simulink model "IEEE30_case"  (R2024b)
settings: Solver=FixedStepAuto  StartTime=0  StopTime=5  FixedStep=1e-7  RelTol=1e-3
values from neighbouring files (symbols this model uses):
  GFL_DFIG_7_C_bus = 0.08    [IEEE30_case_parameters.m]
  GFL_DFIG_7_D_mutual = 2.500000e+3    (= 2500)    [IEEE30_case_parameters.m]
  GFL_DFIG_7_f0 = 60    [IEEE30_case_parameters.m]
  GFL_DFIG_7_gPLLi = 3200    [IEEE30_case_parameters.m]
  GFL_DFIG_7_gPLLp = 650    [IEEE30_case_parameters.m]
  GFL_DFIG_7_H_WT = 0.4    [IEEE30_case_parameters.m]
  GFL_DFIG_7_Hg = 0.8    [IEEE30_case_parameters.m]
  GFL_DFIG_7_Igq_ref = 0    [IEEE30_case_parameters.m]
  GFL_DFIG_7_Ird_ref = 704.45696    [IEEE30_case_parameters.m]
  GFL_DFIG_7_KI_V = -300000    [IEEE30_case_parameters.m]
  GFL_DFIG_7_KP_V = -1000    [IEEE30_case_parameters.m]
  GFL_DFIG_7_Ksh = 1.254300e+4    (= 12543)    [IEEE30_case_parameters.m]
  GFL_DFIG_7_Lg = 0.000483    [IEEE30_case_parameters.m]
  GFL_DFIG_7_Lm_pu = 4    [IEEE30_case_parameters.m]
  GFL_DFIG_7_N = 100    [IEEE30_case_parameters.m]
  GFL_DFIG_7_p = 2    [IEEE30_case_parameters.m]
  GFL_DFIG_7_Pitch = 0    [IEEE30_case_parameters.m]
  GFL_DFIG_7_R = 44    [IEEE30_case_parameters.m]
  GFL_DFIG_7_Rg = 2.000000e-5    (= 2e-05)    [IEEE30_case_parameters.m]
  GFL_DFIG_7_rho = 1.225    [IEEE30_case_parameters.m]
  GFL_DFIG_7_rPLLi = 4500    [IEEE30_case_parameters.m]
  GFL_DFIG_7_rPLLp = 620    [IEEE30_case_parameters.m]
  GFL_DFIG_7_Rs_pu = 0.011    [IEEE30_case_parameters.m]
  GFL_DFIG_7_Sbase = 2.000000e+6    (= 2000000)    [IEEE30_case_parameters.m]
  GFL_DFIG_7_ugq_ref = 0    [IEEE30_case_parameters.m]
  GFL_DFIG_7_usd_ref = 0    [IEEE30_case_parameters.m]
  GFL_DFIG_7_Vbase = 690    [IEEE30_case_parameters.m]
  GFL_DFIG_7_Vdc_ref = 1200    [IEEE30_case_parameters.m]
  GFL_DFIG_7_wind = 12    [IEEE30_case_parameters.m]
  GFL_DFIG_7_wm_ref = 518.184209    [IEEE30_case_parameters.m]
  SG_D_13_D = 0.01056    [IEEE30_case_parameters.m]
  SG_D_13_EnableSaturation = 0    [IEEE30_case_parameters.m]
  SG_D_13_f0 = 60    [IEEE30_case_parameters.m]
  SG_D_13_H = 7.5    [IEEE30_case_parameters.m]
  SG_D_13_K_A = 20    [IEEE30_case_parameters.m]
  SG_D_13_K_E = 1.000000e+1    (= 10)    [IEEE30_case_parameters.m]
  SG_D_13_K_F = 2.363    [IEEE30_case_parameters.m]
  SG_D_13_K_s = 0.5    [IEEE30_case_parameters.m]
  SG_D_13_R_a = 0.001088    [IEEE30_case_parameters.m]
  SG_D_13_S_A = 1    [IEEE30_case_parameters.m]
  SG_D_13_S_B = 0.103    [IEEE30_case_parameters.m]
  SG_D_13_S_N = 10.659857    [IEEE30_case_parameters.m]
  SG_D_13_SpeedPara = 200    [IEEE30_case_parameters.m]
  SG_D_13_T_0 = 0.370163    [IEEE30_case_parameters.m]
  SG_D_13_T_1 = 0.3    [IEEE30_case_parameters.m]
  SG_D_13_T_2 = 0.05    [IEEE30_case_parameters.m]
  SG_D_13_T_3 = 0.02    [IEEE30_case_parameters.m]
  SG_D_13_T_4 = 0.005    [IEEE30_case_parameters.m]
  SG_D_13_T_A = 0.02    [IEEE30_case_parameters.m]
  SG_D_13_T_dd = 8.000000e+0    (= 8)    [IEEE30_case_parameters.m]
  SG_D_13_T_ddd = 0.04    [IEEE30_case_parameters.m]
  SG_D_13_T_E = 0.314    [IEEE30_case_parameters.m]
  SG_D_13_T_F = 0.35    [IEEE30_case_parameters.m]
  SG_D_13_T_qd = 0.8    [IEEE30_case_parameters.m]
  SG_D_13_T_qdd = 0.02    [IEEE30_case_parameters.m]
  SG_D_13_T_speed = 0.1    [IEEE30_case_parameters.m]
  SG_D_13_T_w = 0.5    [IEEE30_case_parameters.m]
  SG_D_13_V_ref = 1.696619    [IEEE30_case_parameters.m]
  SG_D_13_w_ref = 376.991118    [IEEE30_case_parameters.m]
  SG_D_13_x_d = 1.9    [IEEE30_case_parameters.m]
  SG_D_13_x_dd = 0.302    [IEEE30_case_parameters.m]
  SG_D_13_x_ddd = 0.204    [IEEE30_case_parameters.m]
  SG_D_13_x_l = 0.05    [IEEE30_case_parameters.m]
  SG_D_13_x_q = 1.3    [IEEE30_case_parameters.m]
  SG_D_13_x_qd = 0.5    [IEEE30_case_parameters.m]
  SG_D_13_x_qdd = 0.3    [IEEE30_case_parameters.m]
  SG_D_1_D = 0.01056    [IEEE30_case_parameters.m]
  SG_D_1_EnableSaturation = 0    [IEEE30_case_parameters.m]
  SG_D_1_f0 = 60    [IEEE30_case_parameters.m]
  SG_D_1_H = 7.5    [IEEE30_case_parameters.m]
  SG_D_1_K_A = 20    [IEEE30_case_parameters.m]
  SG_D_1_K_E = 1.000000e+1    (= 10)    [IEEE30_case_parameters.m]
  SG_D_1_K_F = 2.363    [IEEE30_case_parameters.m]
  SG_D_1_K_s = 0.5    [IEEE30_case_parameters.m]
  SG_D_1_R_a = 0.001088    [IEEE30_case_parameters.m]
  SG_D_1_S_A = 1    [IEEE30_case_parameters.m]
  SG_D_1_S_B = 0.103    [IEEE30_case_parameters.m]
  SG_D_1_S_N = 10.659857    [IEEE30_case_parameters.m]
  SG_D_1_SpeedPara = 200    [IEEE30_case_parameters.m]
  SG_D_1_T_0 = 0.259812    [IEEE30_case_parameters.m]
  SG_D_1_T_1 = 0.3    [IEEE30_case_parameters.m]
  SG_D_1_T_2 = 0.05    [IEEE30_case_parameters.m]
  SG_D_1_T_3 = 0.02    [IEEE30_case_parameters.m]
  SG_D_1_T_4 = 0.005    [IEEE30_case_parameters.m]
  SG_D_1_T_A = 0.02    [IEEE30_case_parameters.m]
  SG_D_1_T_dd = 8.000000e+0    (= 8)    [IEEE30_case_parameters.m]
  SG_D_1_T_ddd = 0.04    [IEEE30_case_parameters.m]
  SG_D_1_T_E = 0.314    [IEEE30_case_parameters.m]
  SG_D_1_T_F = 0.35    [IEEE30_case_parameters.m]
  SG_D_1_T_qd = 0.8    [IEEE30_case_parameters.m]
  SG_D_1_T_qdd = 0.02    [IEEE30_case_parameters.m]
  SG_D_1_T_speed = 0.1    [IEEE30_case_parameters.m]
  SG_D_1_T_w = 0.5    [IEEE30_case_parameters.m]
  SG_D_1_V_ref = 1.544107    [IEEE30_case_parameters.m]
  SG_D_1_w_ref = 376.991118    [IEEE30_case_parameters.m]
  SG_D_1_x_d = 1.9    [IEEE30_case_parameters.m]
  SG_D_1_x_dd = 0.302    [IEEE30_case_parameters.m]
  SG_D_1_x_ddd = 0.204    [IEEE30_case_parameters.m]
  SG_D_1_x_l = 0.05    [IEEE30_case_parameters.m]
  SG_D_1_x_q = 1.3    [IEEE30_case_parameters.m]
  SG_D_1_x_qd = 0.5    [IEEE30_case_parameters.m]
  SG_D_1_x_qdd = 0.3    [IEEE30_case_parameters.m]
  SG_D_22_D = 0.01056    [IEEE30_case_parameters.m]
  SG_D_22_EnableSaturation = 0    [IEEE30_case_parameters.m]
  SG_D_22_f0 = 60    [IEEE30_case_parameters.m]
  SG_D_22_H = 7.5    [IEEE30_case_parameters.m]
  SG_D_22_K_A = 20    [IEEE30_case_parameters.m]
  SG_D_22_K_E = 1.000000e+1    (= 10)    [IEEE30_case_parameters.m]
  SG_D_22_K_F = 2.363    [IEEE30_case_parameters.m]
  SG_D_22_K_s = 0.5    [IEEE30_case_parameters.m]
  SG_D_22_R_a = 0.001088    [IEEE30_case_parameters.m]
  SG_D_22_S_A = 1    [IEEE30_case_parameters.m]
  SG_D_22_S_B = 0.103    [IEEE30_case_parameters.m]
  SG_D_22_S_N = 10.659857    [IEEE30_case_parameters.m]
  SG_D_22_SpeedPara = 200    [IEEE30_case_parameters.m]
  SG_D_22_T_0 = 0.216121    [IEEE30_case_parameters.m]
  SG_D_22_T_1 = 0.3    [IEEE30_case_parameters.m]
  SG_D_22_T_2 = 0.05    [IEEE30_case_parameters.m]
  SG_D_22_T_3 = 0.02    [IEEE30_case_parameters.m]
  SG_D_22_T_4 = 0.005    [IEEE30_case_parameters.m]
  ... (+126 more)
(part 3 of 27)

== system IEEE30_case/GFL_DFIG_7 ==
  v_d_GFL_DFIG_7 : Inport
  v_q_GFL_DFIG_7 : Inport  Port=2
  Phi_ga_GFL_DFIG_7 : Integrator  InitialCondition=-3.864590758475076e-10
  Phi_gb_GFL_DFIG_7 : Integrator  InitialCondition=0.009328141747306295
  Phi_gc_GFL_DFIG_7 : Integrator  InitialCondition=482731.33548516966
  Phi_ra_GFL_DFIG_7 : Integrator  InitialCondition=2.029121350382751
  Phi_rb_GFL_DFIG_7 : Integrator  InitialCondition=3.675917935843726
  Phi_rc_GFL_DFIG_7 : Integrator  InitialCondition=-6744.715803637379
  Phipllg_GFL_DFIG_7 : Integrator  InitialCondition=0.0
  Phipllr_GFL_DFIG_7 : Integrator  InitialCondition=0.0
  Psi_dr_GFL_DFIG_7 : Integrator  InitialCondition=1.7971026996671524
  Psi_ds_GFL_DFIG_7 : Integrator  InitialCondition=1.7793096036324896
  Psi_qr_GFL_DFIG_7 : Integrator  InitialCondition=0.06414812889743245
  Psi_qs_GFL_DFIG_7 : Integrator  InitialCondition=2.273401543592287e-13
  T_e_GFL_DFIG_7_block : Subsystem
  Turbine_w_GFL_DFIG_7 : Integrator  InitialCondition=259.0921046354467
  V_dc_GFL_DFIG_7 : Integrator  InitialCondition=1200.0
  d_Phi_ga_GFL_DFIG_7_block : Subsystem
  d_Phi_gb_GFL_DFIG_7_block : Subsystem
  d_Phi_gc_GFL_DFIG_7_block : Subsystem
  d_Phi_ra_GFL_DFIG_7_block : Subsystem
  d_Phi_rb_GFL_DFIG_7_block : Subsystem
  d_Phi_rc_GFL_DFIG_7_block : Subsystem
  d_Phipllg_GFL_DFIG_7_block : Subsystem
  d_Phipllr_GFL_DFIG_7_block : Subsystem
  d_Psi_dr_GFL_DFIG_7_block : Subsystem
  d_Psi_ds_GFL_DFIG_7_block : Subsystem
  d_Psi_qr_GFL_DFIG_7_block : Subsystem
  d_Psi_qs_GFL_DFIG_7_block : Subsystem
  d_Turbine_w_GFL_DFIG_7_block : Subsystem
  d_V_dc_GFL_DFIG_7_block : Subsystem
  d_i_gd_GFL_DFIG_7_block : Subsystem
  d_i_gq_GFL_DFIG_7_block : Subsystem
  d_shaft_w_GFL_DFIG_7_block : Subsystem
  d_theta_pllg_GFL_DFIG_7_block : Subsystem
  d_theta_pllr_GFL_DFIG_7_block : Subsystem
  d_w_m_GFL_DFIG_7_block : Subsystem
  i_d_GFL_DFIG_7_block : Subsystem
  i_gd_GFL_DFIG_7 : Integrator  InitialCondition=466.4070874252847
  i_gq_GFL_DFIG_7 : Integrator  InitialCondition=5.309080990232214e-32
  i_q_GFL_DFIG_7_block : Subsystem
  shaft_w_GFL_DFIG_7 : Integrator  InitialCondition=-0.620914212798937
  theta_pllg_GFL_DFIG_7 : Integrator  InitialCondition=0.04628328286195157
  theta_pllr_GFL_DFIG_7 : Integrator  InitialCondition=-1.5245130439329455
  w_m_GFL_DFIG_7 : Integrator  InitialCondition=518.1842092708933
  w_r_GFL_DFIG_7_block : Subsystem
  i_d_GFL_DFIG_7 : Outport
  i_q_GFL_DFIG_7 : Outport  Port=2
  T_e_GFL_DFIG_7 : Outport  Port=3
  w_r_GFL_DFIG_7 : Outport  Port=4
  wires:
  Phipllg_GFL_DFIG_7/1 -> d_theta_pllg_GFL_DFIG_7_block/1(State_Phipllg_GFL_DFIG_7_ae55c)
  d_w_m_GFL_DFIG_7_block/1(Blockout_d_w_m_GFL_DFIG_7_977b5) -> w_m_GFL_DFIG_7/1
  i_gd_GFL_DFIG_7/1 -> d_i_gd_GFL_DFIG_7_block/3(State_i_gd_GFL_DFIG_7_79282), i_q_GFL_DFIG_7_block/1(State_i_gd_GFL_DFIG_7_7f088), i_d_GFL_DFIG_7_block/1(State_i_gd_GFL_DFIG_7_c7c38), d_i_gd_GFL_DFIG_7_block/2(State_i_gd_GFL_DFIG_7_e096c), d_V_dc_GFL_DFIG_7_block/1(State_i_gd_GFL_DFIG_7_47a9f), d_Phi_gb_GFL_DFIG_7_block/1(State_i_gd_GFL_DFIG_7_640f4)
  d_Psi_ds_GFL_DFIG_7_block/1(Blockout_d_Psi_ds_GFL_DFIG_7_0935c) -> Psi_ds_GFL_DFIG_7/1
  Phipllr_GFL_DFIG_7/1 -> d_theta_pllr_GFL_DFIG_7_block/1(State_Phipllr_GFL_DFIG_7_8b535)
  i_d_GFL_DFIG_7_block/1(Blockout_i_d_GFL_DFIG_7_2a8ae) -> i_d_GFL_DFIG_7/1
  d_Psi_qr_GFL_DFIG_7_block/1(Blockout_d_Psi_qr_GFL_DFIG_7_49d19) -> Psi_qr_GFL_DFIG_7/1
  i_q_GFL_DFIG_7_block/1(Blockout_i_q_GFL_DFIG_7_ec3de) -> i_q_GFL_DFIG_7/1
  d_Psi_qs_GFL_DFIG_7_block/1(Blockout_d_Psi_qs_GFL_DFIG_7_2d6b6) -> Psi_qs_GFL_DFIG_7/1
  v_q_GFL_DFIG_7/1 -> d_theta_pllr_GFL_DFIG_7_block/4(Input_v_q_GFL_DFIG_7_cdd0f), d_Phipllr_GFL_DFIG_7_block/3(Input_v_q_GFL_DFIG_7_661f6), d_Psi_qs_GFL_DFIG_7_block/6(Input_v_q_GFL_DFIG_7_1b265), d_theta_pllg_GFL_DFIG_7_block/4(Input_v_q_GFL_DFIG_7_c7c1e), d_Phipllg_GFL_DFIG_7_block/3(Input_v_q_GFL_DFIG_7_4b381), d_Psi_ds_GFL_DFIG_7_block/6(Input_v_q_GFL_DFIG_7_712eb), d_V_dc_GFL_DFIG_7_block/4(Input_v_q_GFL_DFIG_7_3c611), d_V_dc_GFL_DFIG_7_block/9(Input_v_q_GFL_DFIG_7_49107)
  Turbine_w_GFL_DFIG_7/1 -> d_shaft_w_GFL_DFIG_7_block/1(State_Turbine_w_GFL_DFIG_7_fd30f), d_w_m_GFL_DFIG_7_block/1(State_Turbine_w_GFL_DFIG_7_8e651), d_Turbine_w_GFL_DFIG_7_block/5(State_Turbine_w_GFL_DFIG_7_921a6), d_Turbine_w_GFL_DFIG_7_block/6(State_Turbine_w_GFL_DFIG_7_deaae), d_Turbine_w_GFL_DFIG_7_block/4(State_Turbine_w_GFL_DFIG_7_01506), d_Turbine_w_GFL_DFIG_7_block/1(State_Turbine_w_GFL_DFIG_7_f59a7)
  d_V_dc_GFL_DFIG_7_block/1(Blockout_d_V_dc_GFL_DFIG_7_1a7e1) -> V_dc_GFL_DFIG_7/1
  w_r_GFL_DFIG_7_block/1(Blockout_w_r_GFL_DFIG_7_71344) -> w_r_GFL_DFIG_7/1
  theta_pllr_GFL_DFIG_7/1 -> d_theta_pllr_GFL_DFIG_7_block/5(State_theta_pllr_GFL_DFIG_7_76fa6), d_theta_pllr_GFL_DFIG_7_block/3(State_theta_pllr_GFL_DFIG_7_64a08), d_Psi_ds_GFL_DFIG_7_block/7(State_theta_pllr_GFL_DFIG_7_2fe4a), d_Psi_ds_GFL_DFIG_7_block/5(State_theta_pllr_GFL_DFIG_7_d96f9), d_Phipllr_GFL_DFIG_7_block/2(State_theta_pllr_GFL_DFIG_7_673d7), d_Phipllr_GFL_DFIG_7_block/4(State_theta_pllr_GFL_DFIG_7_c3596), i_q_GFL_DFIG_7_block/10(State_theta_pllr_GFL_DFIG_7_b0808), d_Psi_qs_GFL_DFIG_7_block/5(State_theta_pllr_GFL_DFIG_7_5db89), d_Psi_qs_GFL_DFIG_7_block/7(State_theta_pllr_GFL_DFIG_7_ab88b), i_d_GFL_DFIG_7_block/7(State_theta_pllr_GFL_DFIG_7_79db7), i_d_GFL_DFIG_7_block/10(State_theta_pllr_GFL_DFIG_7_e04ad), i_q_GFL_DFIG_7_block/7(State_theta_pllr_GFL_DFIG_7_9bdbf)
  V_dc_GFL_DFIG_7/1 -> d_Phi_gc_GFL_DFIG_7_block/1(State_V_dc_GFL_DFIG_7_30c65), d_i_gd_GFL_DFIG_7_block/4(State_V_dc_GFL_DFIG_7_27989), d_Phi_gb_GFL_DFIG_7_block/2(State_V_dc_GFL_DFIG_7_6d222), d_V_dc_GFL_DFIG_7_block/34(State_V_dc_GFL_DFIG_7_49932)
  Phi_ga_GFL_DFIG_7/1 -> d_i_gq_GFL_DFIG_7_block/1(State_Phi_ga_GFL_DFIG_7_1abf4)
  T_e_GFL_DFIG_7_block/1(Blockout_T_e_GFL_DFIG_7_ea981) -> T_e_GFL_DFIG_7/1
  Phi_gb_GFL_DFIG_7/1 -> d_i_gd_GFL_DFIG_7_block/1(State_Phi_gb_GFL_DFIG_7_1acd8)
  d_Phipllg_GFL_DFIG_7_block/1(Blockout_d_Phipllg_GFL_DFIG_7_57d75) -> Phipllg_GFL_DFIG_7/1
  theta_pllg_GFL_DFIG_7/1 -> d_theta_pllg_GFL_DFIG_7_block/3(State_theta_pllg_GFL_DFIG_7_2f4db), d_theta_pllg_GFL_DFIG_7_block/5(State_theta_pllg_GFL_DFIG_7_b3c0b), i_d_GFL_DFIG_7_block/2(State_theta_pllg_GFL_DFIG_7_3c4e6), i_d_GFL_DFIG_7_block/4(State_theta_pllg_GFL_DFIG_7_99cce), i_q_GFL_DFIG_7_block/2(State_theta_pllg_GFL_DFIG_7_b67ea), i_q_GFL_DFIG_7_block/4(State_theta_pllg_GFL_DFIG_7_36f0a), d_Phipllg_GFL_DFIG_7_block/4(State_theta_pllg_GFL_DFIG_7_1f5b3), d_Phipllg_GFL_DFIG_7_block/2(State_theta_pllg_GFL_DFIG_7_d7c88), d_V_dc_GFL_DFIG_7_block/3(State_theta_pllg_GFL_DFIG_7_c67a2), d_V_dc_GFL_DFIG_7_block/5(State_theta_pllg_GFL_DFIG_7_35391), d_V_dc_GFL_DFIG_7_block/8(State_theta_pllg_GFL_DFIG_7_002e2), d_V_dc_GFL_DFIG_7_block/10(State_theta_pllg_GFL_DFIG_7_66e51)
  i_gq_GFL_DFIG_7/1 -> d_i_gq_GFL_DFIG_7_block/3(State_i_gq_GFL_DFIG_7_5be6d), d_i_gq_GFL_DFIG_7_block/2(State_i_gq_GFL_DFIG_7_3f6ab), d_Phi_ga_GFL_DFIG_7_block/1(State_i_gq_GFL_DFIG_7_ca300), i_q_GFL_DFIG_7_block/3(State_i_gq_GFL_DFIG_7_cf5eb), d_V_dc_GFL_DFIG_7_block/6(State_i_gq_GFL_DFIG_7_793b6), i_d_GFL_DFIG_7_block/3(State_i_gq_GFL_DFIG_7_12231)
  d_Phipllr_GFL_DFIG_7_block/1(Blockout_d_Phipllr_GFL_DFIG_7_3fa24) -> Phipllr_GFL_DFIG_7/1
  Psi_qs_GFL_DFIG_7/1 -> T_e_GFL_DFIG_7_block/4(State_Psi_qs_GFL_DFIG_7_92c6b), T_e_GFL_DFIG_7_block/8(State_Psi_qs_GFL_DFIG_7_3687d), d_Psi_dr_GFL_DFIG_7_block/3(State_Psi_qs_GFL_DFIG_7_a7547), d_Psi_qr_GFL_DFIG_7_block/16(State_Psi_qs_GFL_DFIG_7_c351a), i_d_GFL_DFIG_7_block/9(State_Psi_qs_GFL_DFIG_7_a1324), d_Phi_rb_GFL_DFIG_7_block/4(State_Psi_qs_GFL_DFIG_7_57503), d_Phi_rb_GFL_DFIG_7_block/6(State_Psi_qs_GFL_DFIG_7_e35cc), i_q_GFL_DFIG_7_block/9(State_Psi_qs_GFL_DFIG_7_79723), d_w_m_GFL_DFIG_7_block/7(State_Psi_qs_GFL_DFIG_7_716ac), d_w_m_GFL_DFIG_7_block/11(State_Psi_qs_GFL_DFIG_7_6b007), d_Psi_ds_GFL_DFIG_7_block/1(State_Psi_qs_GFL_DFIG_7_b4caa), d_Psi_qr_GFL_DFIG_7_block/8(State_Psi_qs_GFL_DFIG_7_981a4), d_Psi_qr_GFL_DFIG_7_block/12(State_Psi_qs_GFL_DFIG_7_b24c8), d_Psi_qr_GFL_DFIG_7_block/14(State_Psi_qs_GFL_DFIG_7_c0308), d_Psi_qs_GFL_DFIG_7_block/3(State_Psi_qs_GFL_DFIG_7_b8433), d_V_dc_GFL_DFIG_7_block/30(State_Psi_qs_GFL_DFIG_7_44146), d_V_dc_GFL_DFIG_7_block/32(State_Psi_qs_GFL_DFIG_7_97bd8), d_V_dc_GFL_DFIG_7_block/28(State_Psi_qs_GFL_DFIG_7_f7902), d_V_dc_GFL_DFIG_7_block/20(State_Psi_qs_GFL_DFIG_7_fde33), d_V_dc_GFL_DFIG_7_block/15(State_Psi_qs_GFL_DFIG_7_f70b4)
  d_Phi_gb_GFL_DFIG_7_block/1(Blockout_d_Phi_gb_GFL_DFIG_7_12bfd) -> Phi_gb_GFL_DFIG_7/1
  d_Phi_gc_GFL_DFIG_7_block/1(Blockout_d_Phi_gc_GFL_DFIG_7_e7a32) -> Phi_gc_GFL_DFIG_7/1
  d_Phi_ga_GFL_DFIG_7_block/1(Blockout_d_Phi_ga_GFL_DFIG_7_179fc) -> Phi_ga_GFL_DFIG_7/1
  Psi_dr_GFL_DFIG_7/1 -> d_Psi_dr_GFL_DFIG_7_block/9(State_Psi_dr_GFL_DFIG_7_ac80b), d_Psi_dr_GFL_DFIG_7_block/7(State_Psi_dr_GFL_DFIG_7_f20f7), d_V_dc_GFL_DFIG_7_block/22(State_Psi_dr_GFL_DFIG_7_978cf), d_V_dc_GFL_DFIG_7_block/17(State_Psi_dr_GFL_DFIG_7_0acea), d_V_dc_GFL_DFIG_7_block/11(State_Psi_dr_GFL_DFIG_7_6e653), T_e_GFL_DFIG_7_block/1(State_Psi_dr_GFL_DFIG_7_7f61d), T_e_GFL_DFIG_7_block/5(State_Psi_dr_GFL_DFIG_7_e7cd2), i_d_GFL_DFIG_7_block/5(State_Psi_dr_GFL_DFIG_7_47f96), d_Phi_ra_GFL_DFIG_7_block/1(State_Psi_dr_GFL_DFIG_7_3e6d6), i_q_GFL_DFIG_7_block/5(State_Psi_dr_GFL_DFIG_7_f818d), d_Psi_qr_GFL_DFIG_7_block/5(State_Psi_dr_GFL_DFIG_7_851ca), d_Psi_qr_GFL_DFIG_7_block/2(State_Psi_dr_GFL_DFIG_7_54fa3), d_Psi_ds_GFL_DFIG_7_block/2(State_Psi_dr_GFL_DFIG_7_0949a), d_w_m_GFL_DFIG_7_block/8(State_Psi_dr_GFL_DFIG_7_9aecf), d_w_m_GFL_DFIG_7_block/4(State_Psi_dr_GFL_DFIG_7_d08b0)
  d_theta_pllg_GFL_DFIG_7_block/1(Blockout_d_theta_pllg_GFL_DFIG_7_9b0fc) -> theta_pllg_GFL_DFIG_7/1
  Phi_gc_GFL_DFIG_7/1 -> d_i_gd_GFL_DFIG_7_block/5(State_Phi_gc_GFL_DFIG_7_ffb8d), d_Phi_gb_GFL_DFIG_7_block/3(State_Phi_gc_GFL_DFIG_7_b7107)
  d_theta_pllr_GFL_DFIG_7_block/1(Blockout_d_theta_pllr_GFL_DFIG_7_2facc) -> theta_pllr_GFL_DFIG_7/1
  d_Phi_rb_GFL_DFIG_7_block/1(Blockout_d_Phi_rb_GFL_DFIG_7_7ae6c) -> Phi_rb_GFL_DFIG_7/1
  d_Psi_dr_GFL_DFIG_7_block/1(Blockout_d_Psi_dr_GFL_DFIG_7_75b07) -> Psi_dr_GFL_DFIG_7/1
  d_Phi_rc_GFL_DFIG_7_block/1(Blockout_d_Phi_rc_GFL_DFIG_7_aa447) -> Phi_rc_GFL_DFIG_7/1
  Phi_rc_GFL_DFIG_7/1 -> d_Psi_qr_GFL_DFIG_7_block/9(State_Phi_rc_GFL_DFIG_7_1cf80), d_Phi_rb_GFL_DFIG_7_block/1(State_Phi_rc_GFL_DFIG_7_bc2c9), d_V_dc_GFL_DFIG_7_block/25(State_Phi_rc_GFL_DFIG_7_c7d1c)
  d_Phi_ra_GFL_DFIG_7_block/1(Blockout_d_Phi_ra_GFL_DFIG_7_b9bb2) -> Phi_ra_GFL_DFIG_7/1
  d_Turbine_w_GFL_DFIG_7_block/1(Blockout_d_Turbine_w_GFL_DFIG_7_37f45) -> Turbine_w_GFL_DFIG_7/1
  v_d_GFL_DFIG_7/1 -> d_theta_pllr_GFL_DFIG_7_block/2(Input_v_d_GFL_DFIG_7_57b0c), d_Phipllr_GFL_DFIG_7_block/1(Input_v_d_GFL_DFIG_7_0a8be), d_theta_pllg_GFL_DFIG_7_block/2(Input_v_d_GFL_DFIG_7_973c5), d_Phipllg_GFL_DFIG_7_block/1(Input_v_d_GFL_DFIG_7_9bb07), d_Psi_ds_GFL_DFIG_7_block/4(Input_v_d_GFL_DFIG_7_61464), d_Psi_qs_GFL_DFIG_7_block/4(Input_v_d_GFL_DFIG_7_b1351), d_V_dc_GFL_DFIG_7_block/2(Input_v_d_GFL_DFIG_7_58356), d_V_dc_GFL_DFIG_7_block/7(Input_v_d_GFL_DFIG_7_bbd62)
  w_m_GFL_DFIG_7/1 -> d_Psi_dr_GFL_DFIG_7_block/1(State_w_m_GFL_DFIG_7_ede24), d_Psi_dr_GFL_DFIG_7_block/6(State_w_m_GFL_DFIG_7_c0fab), w_r_GFL_DFIG_7_block/1(State_w_m_GFL_DFIG_7_cf772), d_V_dc_GFL_DFIG_7_block/33(State_w_m_GFL_DFIG_7_46811), d_V_dc_GFL_DFIG_7_block/26(State_w_m_GFL_DFIG_7_35e3b), d_V_dc_GFL_DFIG_7_block/21(State_w_m_GFL_DFIG_7_73a6c), d_V_dc_GFL_DFIG_7_block/13(State_w_m_GFL_DFIG_7_6ca23), d_Psi_qr_GFL_DFIG_7_block/10(State_w_m_GFL_DFIG_7_509a1), d_Phi_rc_GFL_DFIG_7_block/1(State_w_m_GFL_DFIG_7_b5946), d_Psi_qr_GFL_DFIG_7_block/6(State_w_m_GFL_DFIG_7_7741f), d_Psi_qr_GFL_DFIG_7_block/1(State_w_m_GFL_DFIG_7_5fc1b), d_shaft_w_GFL_DFIG_7_block/2(State_w_m_GFL_DFIG_7_93de0), d_w_m_GFL_DFIG_7_block/2(State_w_m_GFL_DFIG_7_dfde2), d_Turbine_w_GFL_DFIG_7_block/2(State_w_m_GFL_DFIG_7_7a0a3), d_Psi_qr_GFL_DFIG_7_block/17(State_w_m_GFL_DFIG_7_084b2), d_Phi_rb_GFL_DFIG_7_block/2(State_w_m_GFL_DFIG_7_5425d)
  Psi_qr_GFL_DFIG_7/1 -> d_Psi_dr_GFL_DFIG_7_block/2(State_Psi_qr_GFL_DFIG_7_b0873), d_Psi_dr_GFL_DFIG_7_block/5(State_Psi_qr_GFL_DFIG_7_8feb7), T_e_GFL_DFIG_7_block/7(State_Psi_qr_GFL_DFIG_7_aa7be), T_e_GFL_DFIG_7_block/3(State_Psi_qr_GFL_DFIG_7_3f5fe), d_Psi_qs_GFL_DFIG_7_block/2(State_Psi_qr_GFL_DFIG_7_e0b4f), d_w_m_GFL_DFIG_7_block/6(State_Psi_qr_GFL_DFIG_7_240a6), i_q_GFL_DFIG_7_block/8(State_Psi_qr_GFL_DFIG_7_bf209), d_w_m_GFL_DFIG_7_block/10(State_Psi_qr_GFL_DFIG_7_28155), i_d_GFL_DFIG_7_block/8(State_Psi_qr_GFL_DFIG_7_2c5a7), d_V_dc_GFL_DFIG_7_block/14(State_Psi_qr_GFL_DFIG_7_2b0e8), d_V_dc_GFL_DFIG_7_block/19(State_Psi_qr_GFL_DFIG_7_f1f75), d_V_dc_GFL_DFIG_7_block/29(State_Psi_qr_GFL_DFIG_7_e69a0), d_Psi_qr_GFL_DFIG_7_block/7(State_Psi_qr_GFL_DFIG_7_c4d86), d_Psi_qr_GFL_DFIG_7_block/13(State_Psi_qr_GFL_DFIG_7_7bb62), d_Phi_rb_GFL_DFIG_7_block/5(State_Psi_qr_GFL_DFIG_7_e4388)
  Psi_ds_GFL_DFIG_7/1 -> d_Psi_dr_GFL_DFIG_7_block/8(State_Psi_ds_GFL_DFIG_7_ccb41), d_Psi_dr_GFL_DFIG_7_block/10(State_Psi_ds_GFL_DFIG_7_652d4), T_e_GFL_DFIG_7_block/6(State_Psi_ds_GFL_DFIG_7_ef1b2), T_e_GFL_DFIG_7_block/2(State_Psi_ds_GFL_DFIG_7_93139), d_Phi_ra_GFL_DFIG_7_block/2(State_Psi_ds_GFL_DFIG_7_9adb5), d_w_m_GFL_DFIG_7_block/5(State_Psi_ds_GFL_DFIG_7_b9ddc), i_q_GFL_DFIG_7_block/6(State_Psi_ds_GFL_DFIG_7_97cbe), d_w_m_GFL_DFIG_7_block/9(State_Psi_ds_GFL_DFIG_7_7aea2), i_d_GFL_DFIG_7_block/6(State_Psi_ds_GFL_DFIG_7_8722f), d_Phi_rb_GFL_DFIG_7_block/3(State_Psi_ds_GFL_DFIG_7_7a16b), d_V_dc_GFL_DFIG_7_block/12(State_Psi_ds_GFL_DFIG_7_832af), d_V_dc_GFL_DFIG_7_block/18(State_Psi_ds_GFL_DFIG_7_692c3), d_V_dc_GFL_DFIG_7_block/23(State_Psi_ds_GFL_DFIG_7_2e09c), d_V_dc_GFL_DFIG_7_block/31(State_Psi_ds_GFL_DFIG_7_a0019), d_V_dc_GFL_DFIG_7_block/27(State_Psi_ds_GFL_DFIG_7_dee5b), d_Psi_qs_GFL_DFIG_7_block/1(State_Psi_ds_GFL_DFIG_7_90de9), d_Psi_ds_GFL_DFIG_7_block/3(State_Psi_ds_GFL_DFIG_7_d7878), d_Psi_qr_GFL_DFIG_7_block/3(State_Psi_ds_GFL_DFIG_7_18bf4), d_Psi_qr_GFL_DFIG_7_block/11(State_Psi_ds_GFL_DFIG_7_e95d8), d_Psi_qr_GFL_DFIG_7_block/15(State_Psi_ds_GFL_DFIG_7_fa3e8)
  shaft_w_GFL_DFIG_7/1 -> d_w_m_GFL_DFIG_7_block/3(State_shaft_w_GFL_DFIG_7_e1a06), d_Turbine_w_GFL_DFIG_7_block/3(State_shaft_w_GFL_DFIG_7_53793)
  Phi_ra_GFL_DFIG_7/1 -> d_Psi_dr_GFL_DFIG_7_block/4(State_Phi_ra_GFL_DFIG_7_e382b), d_V_dc_GFL_DFIG_7_block/16(State_Phi_ra_GFL_DFIG_7_71e34)
  Phi_rb_GFL_DFIG_7/1 -> d_Psi_qr_GFL_DFIG_7_block/4(State_Phi_rb_GFL_DFIG_7_b6830), d_V_dc_GFL_DFIG_7_block/24(State_Phi_rb_GFL_DFIG_7_e2f9d)
  d_i_gd_GFL_DFIG_7_block/1(Blockout_d_i_gd_GFL_DFIG_7_cd2cb) -> i_gd_GFL_DFIG_7/1
  d_i_gq_GFL_DFIG_7_block/1(Blockout_d_i_gq_GFL_DFIG_7_79c3a) -> i_gq_GFL_DFIG_7/1
  d_shaft_w_GFL_DFIG_7_block/1(Blockout_d_shaft_w_GFL_DFIG_7_0b709) -> shaft_w_GFL_DFIG_7/1

== system IEEE30_case/SG_D_1 ==
  v_d_SG_D_1 : Inport
  v_q_SG_D_1 : Inport  Port=2
  E_fd_SG_D_1 : Integrator  InitialCondition=1.0882132920517957
  Px_1_SG_D_1 : Integrator  InitialCondition=0.0
  Px_2_SG_D_1 : Integrator  InitialCondition=0.0
  Px_3_SG_D_1 : Integrator  InitialCondition=-1.2192692551246703e-31
  R_f_SG_D_1 : Integrator  InitialCondition=7.346994311766839
  T_e_SG_D_1_block : Subsystem
  T_m_SG_D_1 : Integrator  InitialCondition=0.2598115405337171
  V_f_SG_D_1 : Integrator  InitialCondition=10.882132920517959
  d_E_fd_SG_D_1_block : Subsystem
  d_Px_1_SG_D_1_block : Subsystem
  d_Px_2_SG_D_1_block : Subsystem
  d_Px_3_SG_D_1_block : Subsystem
  d_R_f_SG_D_1_block : Subsystem
  d_T_m_SG_D_1_block : Subsystem
  d_V_f_SG_D_1_block : Subsystem
  d_psi_1d_SG_D_1_block : Subsystem
  d_psi_d_SG_D_1_block : Subsystem
  d_psi_fd_SG_D_1_block : Subsystem
  d_psi_gq_SG_D_1_block : Subsystem
  d_psi_kq_SG_D_1_block : Subsystem
  d_psi_q_SG_D_1_block : Subsystem
  d_theta_SG_D_1_block : Subsystem
  d_w_SG_D_1_block : Subsystem
  i_d_SG_D_1_block : Subsystem
  i_q_SG_D_1_block : Subsystem
  psi_1d_SG_D_1 : Integrator  InitialCondition=0.950191905636144
  psi_d_SG_D_1 : Integrator  InitialCondition=0.9464615978951803
  psi_fd_SG_D_1 : Integrator  InitialCondition=0.9689926566506003
  psi_gq_SG_D_1 : Integrator  InitialCondition=0.1991943191066703
  psi_kq_SG_D_1 : Integrator  InitialCondition=-0.31124112360417233
  psi_q_SG_D_1 : Integrator  InitialCondition=-0.3236907685483392
  theta_SG_D_1 : Integrator  InitialCondition=0.32954188376716115
  theta_SG_D_1_out_block : Subsystem
  w_SG_D_1 : Integrator  InitialCondition=376.99111843077515
  w_SG_D_1_out_block : Subsystem
  i_d_SG_D_1 : Outport
  i_q_SG_D_1 : Outport  Port=2
  T_e_SG_D_1 : Outport  Port=3
  w_SG_D_1_out : Outport  Port=4
  theta_SG_D_1_out : Outport  Port=5
  wires:
  d_theta_SG_D_1_block/1(Blockout_d_theta_SG_D_1_b4601) -> theta_SG_D_1/1
  d_Px_1_SG_D_1_block/1(Blockout_d_Px_1_SG_D_1_1380a) -> Px_1_SG_D_1/1
  V_f_SG_D_1/1 -> d_V_f_SG_D_1_block/14(State_V_f_SG_D_1_2c940), d_E_fd_SG_D_1_block/2(State_V_f_SG_D_1_4243a)
  psi_kq_SG_D_1/1 -> d_psi_q_SG_D_1_block/2(State_psi_kq_SG_D_1_f77dd), d_psi_gq_SG_D_1_block/3(State_psi_kq_SG_D_1_13d6b), d_psi_gq_SG_D_1_block/5(State_psi_kq_SG_D_1_4933d), d_psi_kq_SG_D_1_block/4(State_psi_kq_SG_D_1_b2a24), d_psi_kq_SG_D_1_block/2(State_psi_kq_SG_D_1_f6edb), d_V_f_SG_D_1_block/10(State_psi_kq_SG_D_1_e81ac), i_d_SG_D_1_block/2(State_psi_kq_SG_D_1_4ef53), d_psi_gq_SG_D_1_block/8(State_psi_kq_SG_D_1_372ae), i_q_SG_D_1_block/2(State_psi_kq_SG_D_1_e6fa4), T_e_SG_D_1_block/3(State_psi_kq_SG_D_1_16b29), d_w_SG_D_1_block/5(State_psi_kq_SG_D_1_2014b)
  w_SG_D_1_out_block/1(Blockout_w_SG_D_1_out_e1973) -> w_SG_D_1_out/1
  w_SG_D_1/1 -> d_psi_d_SG_D_1_block/9(State_w_SG_D_1_d2cfd), d_w_SG_D_1_block/1(State_w_SG_D_1_7370e), d_psi_q_SG_D_1_block/9(State_w_SG_D_1_948ae), d_V_f_SG_D_1_block/8(State_w_SG_D_1_25f13), d_T_m_SG_D_1_block/1(State_w_SG_D_1_e56b0), d_Px_1_SG_D_1_block/2(State_w_SG_D_1_e905d), d_Px_2_SG_D_1_block/4(State_w_SG_D_1_34181), d_Px_3_SG_D_1_block/6(State_w_SG_D_1_e8e94), d_V_f_SG_D_1_block/13(State_w_SG_D_1_84be6), w_SG_D_1_out_block/1(State_w_SG_D_1_f54e8), d_theta_SG_D_1_block/1(State_w_SG_D_1_25fe5)
  d_T_m_SG_D_1_block/1(Blockout_d_T_m_SG_D_1_12514) -> T_m_SG_D_1/1
  d_Px_2_SG_D_1_block/1(Blockout_d_Px_2_SG_D_1_8ee22) -> Px_2_SG_D_1/1
  d_Px_3_SG_D_1_block/1(Blockout_d_Px_3_SG_D_1_3bf99) -> Px_3_SG_D_1/1
  psi_gq_SG_D_1/1 -> d_psi_q_SG_D_1_block/1(State_psi_gq_SG_D_1_26e24), d_psi_gq_SG_D_1_block/1(State_psi_gq_SG_D_1_332f7), d_psi_gq_SG_D_1_block/2(State_psi_gq_SG_D_1_b0dac), d_w_SG_D_1_block/4(State_psi_gq_SG_D_1_ce49a), d_psi_kq_SG_D_1_block/1(State_psi_gq_SG_D_1_66a42), d_V_f_SG_D_1_block/9(State_psi_gq_SG_D_1_d56db), d_psi_kq_SG_D_1_block/3(State_psi_gq_SG_D_1_3bf06), i_d_SG_D_1_block/1(State_psi_gq_SG_D_1_10f28), d_psi_gq_SG_D_1_block/7(State_psi_gq_SG_D_1_3b2a6), d_psi_gq_SG_D_1_block/4(State_psi_gq_SG_D_1_2cb53), i_q_SG_D_1_block/1(State_psi_gq_SG_D_1_d4375), T_e_SG_D_1_block/2(State_psi_gq_SG_D_1_a6910)
  psi_fd_SG_D_1/1 -> d_psi_fd_SG_D_1_block/2(State_psi_fd_SG_D_1_c7574), d_psi_fd_SG_D_1_block/4(State_psi_fd_SG_D_1_fe3bf), d_psi_fd_SG_D_1_block/7(State_psi_fd_SG_D_1_1eed0), d_psi_d_SG_D_1_block/3(State_psi_fd_SG_D_1_f658e), d_psi_1d_SG_D_1_block/2(State_psi_fd_SG_D_1_697dc), i_d_SG_D_1_block/7(State_psi_fd_SG_D_1_0507a), d_psi_1d_SG_D_1_block/5(State_psi_fd_SG_D_1_a7ee9), i_q_SG_D_1_block/7(State_psi_fd_SG_D_1_d5158), T_e_SG_D_1_block/8(State_psi_fd_SG_D_1_a9978), d_w_SG_D_1_block/10(State_psi_fd_SG_D_1_cb4ff), d_V_f_SG_D_1_block/6(State_psi_fd_SG_D_1_18250), d_psi_fd_SG_D_1_block/10(State_psi_fd_SG_D_1_e31c3)
  T_m_SG_D_1/1 -> d_T_m_SG_D_1_block/2(State_T_m_SG_D_1_eb6d8), d_w_SG_D_1_block/2(State_T_m_SG_D_1_0f890)
  v_d_SG_D_1/1 -> d_psi_d_SG_D_1_block/4(Input_v_d_SG_D_1_95be5), d_psi_q_SG_D_1_block/4(Input_v_d_SG_D_1_1c698)
  v_q_SG_D_1/1 -> d_psi_d_SG_D_1_block/6(Input_v_q_SG_D_1_f5767), d_psi_q_SG_D_1_block/6(Input_v_q_SG_D_1_e75ba)
  Px_1_SG_D_1/1 -> d_Px_1_SG_D_1_block/1(State_Px_1_SG_D_1_b81ac), d_Px_3_SG_D_1_block/5(State_Px_1_SG_D_1_665ee), d_Px_3_SG_D_1_block/4(State_Px_1_SG_D_1_64472), d_Px_2_SG_D_1_block/3(State_Px_1_SG_D_1_3856c), d_Px_2_SG_D_1_block/2(State_Px_1_SG_D_1_ae78a)
  Px_2_SG_D_1/1 -> d_Px_2_SG_D_1_block/1(State_Px_2_SG_D_1_7ad78), d_Px_3_SG_D_1_block/2(State_Px_2_SG_D_1_d9b49), d_Px_3_SG_D_1_block/3(State_Px_2_SG_D_1_ab48e)
  theta_SG_D_1/1 -> d_psi_d_SG_D_1_block/5(State_theta_SG_D_1_3e828), d_psi_d_SG_D_1_block/7(State_theta_SG_D_1_93c49), d_psi_q_SG_D_1_block/5(State_theta_SG_D_1_9525e), i_d_SG_D_1_block/4(State_theta_SG_D_1_e11c7), i_d_SG_D_1_block/8(State_theta_SG_D_1_02fe0), i_q_SG_D_1_block/4(State_theta_SG_D_1_9797a), i_q_SG_D_1_block/8(State_theta_SG_D_1_8458a), d_psi_q_SG_D_1_block/7(State_theta_SG_D_1_5ff34), theta_SG_D_1_out_block/1(State_theta_SG_D_1_a2930)
  d_E_fd_SG_D_1_block/1(Blockout_d_E_fd_SG_D_1_3912e) -> E_fd_SG_D_1/1
  psi_1d_SG_D_1/1 -> d_psi_fd_SG_D_1_block/5(State_psi_1d_SG_D_1_b3018), d_psi_fd_SG_D_1_block/8(State_psi_1d_SG_D_1_10652), d_psi_fd_SG_D_1_block/3(State_psi_1d_SG_D_1_1742e), d_psi_d_SG_D_1_block/1(State_psi_1d_SG_D_1_5396e), d_psi_1d_SG_D_1_block/1(State_psi_1d_SG_D_1_acde6), d_psi_1d_SG_D_1_block/3(State_psi_1d_SG_D_1_d153a), i_q_SG_D_1_block/5(State_psi_1d_SG_D_1_a42f8), d_V_f_SG_D_1_block/4(State_psi_1d_SG_D_1_39760), T_e_SG_D_1_block/6(State_psi_1d_SG_D_1_d6542), i_d_SG_D_1_block/5(State_psi_1d_SG_D_1_3ebc3), d_w_SG_D_1_block/8(State_psi_1d_SG_D_1_f2003)
  psi_q_SG_D_1/1 -> d_psi_d_SG_D_1_block/8(State_psi_q_SG_D_1_efd17), d_psi_q_SG_D_1_block/3(State_psi_q_SG_D_1_070ab), d_psi_gq_SG_D_1_block/6(State_psi_q_SG_D_1_31e6a), d_psi_gq_SG_D_1_block/9(State_psi_q_SG_D_1_64712), d_psi_kq_SG_D_1_block/5(State_psi_q_SG_D_1_f72b4), d_V_f_SG_D_1_block/7(State_psi_q_SG_D_1_71447), d_w_SG_D_1_block/7(State_psi_q_SG_D_1_91429), d_w_SG_D_1_block/6(State_psi_q_SG_D_1_d909e), i_q_SG_D_1_block/3(State_psi_q_SG_D_1_6d2ce), T_e_SG_D_1_block/4(State_psi_q_SG_D_1_15adc), d_V_f_SG_D_1_block/11(State_psi_q_SG_D_1_54025), i_d_SG_D_1_block/3(State_psi_q_SG_D_1_228eb), T_e_SG_D_1_block/5(State_psi_q_SG_D_1_53812)
  psi_d_SG_D_1/1 -> d_psi_fd_SG_D_1_block/6(State_psi_d_SG_D_1_a13b4), d_psi_fd_SG_D_1_block/9(State_psi_d_SG_D_1_482bf), d_psi_d_SG_D_1_block/2(State_psi_d_SG_D_1_d85a6), d_psi_q_SG_D_1_block/8(State_psi_d_SG_D_1_80a58), d_w_SG_D_1_block/9(State_psi_d_SG_D_1_182c7), d_V_f_SG_D_1_block/5(State_psi_d_SG_D_1_bcc6e), d_w_SG_D_1_block/3(State_psi_d_SG_D_1_f033d), d_V_f_SG_D_1_block/12(State_psi_d_SG_D_1_40cd3), T_e_SG_D_1_block/1(State_psi_d_SG_D_1_f3ca8), i_d_SG_D_1_block/6(State_psi_d_SG_D_1_fb11e), T_e_SG_D_1_block/7(State_psi_d_SG_D_1_e6af8), d_psi_1d_SG_D_1_block/4(State_psi_d_SG_D_1_ee12b), i_q_SG_D_1_block/6(State_psi_d_SG_D_1_00c64)
  d_psi_gq_SG_D_1_block/1(Blockout_d_psi_gq_SG_D_1_8e30a) -> psi_gq_SG_D_1/1
  d_psi_kq_SG_D_1_block/1(Blockout_d_psi_kq_SG_D_1_05b7c) -> psi_kq_SG_D_1/1
  d_w_SG_D_1_block/1(Blockout_d_w_SG_D_1_18f98) -> w_SG_D_1/1
  d_R_f_SG_D_1_block/1(Blockout_d_R_f_SG_D_1_cb206) -> R_f_SG_D_1/1
  T_e_SG_D_1_block/1(Blockout_T_e_SG_D_1_09252) -> T_e_SG_D_1/1
  d_V_f_SG_D_1_block/1(Blockout_d_V_f_SG_D_1_691ea) -> V_f_SG_D_1/1
  d_psi_q_SG_D_1_block/1(Blockout_d_psi_q_SG_D_1_abfd1) -> psi_q_SG_D_1/1
  d_psi_d_SG_D_1_block/1(Blockout_d_psi_d_SG_D_1_2866c) -> psi_d_SG_D_1/1
  i_q_SG_D_1_block/1(Blockout_i_q_SG_D_1_159c7) -> i_q_SG_D_1/1
  i_d_SG_D_1_block/1(Blockout_i_d_SG_D_1_f91f6) -> i_d_SG_D_1/1
  d_psi_1d_SG_D_1_block/1(Blockout_d_psi_1d_SG_D_1_c059e) -> psi_1d_SG_D_1/1
  theta_SG_D_1_out_block/1(Blockout_theta_SG_D_1_out_f6ef7) -> theta_SG_D_1_out/1
  Px_3_SG_D_1/1 -> d_V_f_SG_D_1_block/3(State_Px_3_SG_D_1_b7bc3), d_Px_3_SG_D_1_block/1(State_Px_3_SG_D_1_caa78)
  R_f_SG_D_1/1 -> d_V_f_SG_D_1_block/2(State_R_f_SG_D_1_57c1d), d_R_f_SG_D_1_block/2(State_R_f_SG_D_1_11fa9)
  E_fd_SG_D_1/1 -> d_V_f_SG_D_1_block/1(State_E_fd_SG_D_1_41419), d_E_fd_SG_D_1_block/1(State_E_fd_SG_D_1_d0430), d_R_f_SG_D_1_block/1(State_E_fd_SG_D_1_7bfd0), d_psi_fd_SG_D_1_block/1(State_E_fd_SG_D_1_d5aee)
  d_psi_fd_SG_D_1_block/1(Blockout_d_psi_fd_SG_D_1_f96ae) -> psi_fd_SG_D_1/1

== system IEEE30_case/SG_D_13 ==
  v_d_SG_D_13 : Inport
  v_q_SG_D_13 : Inport  Port=2
  E_fd_SG_D_13 : Integrator  InitialCondition=1.3932372292894462
  Px_1_SG_D_13 : Integrator  InitialCondition=0.0
  Px_2_SG_D_13 : Integrator  InitialCondition=0.0
  Px_3_SG_D_13 : Integrator  InitialCondition=6.565954607247441e-26
  R_f_SG_D_13 : Integrator  InitialCondition=9.406341636602747
  T_e_SG_D_13_block : Subsystem
  T_m_SG_D_13 : Integrator  InitialCondition=0.3701629699708787
  V_f_SG_D_13 : Integrator  InitialCondition=13.932372292894462
  d_E_fd_SG_D_13_block : Subsystem
  d_Px_1_SG_D_13_block : Subsystem
  d_Px_2_SG_D_13_block : Subsystem
  d_Px_3_SG_D_13_block : Subsystem
  d_R_f_SG_D_13_block : Subsystem
  d_T_m_SG_D_13_block : Subsystem
  d_V_f_SG_D_13_block : Subsystem
  d_psi_1d_SG_D_13_block : Subsystem
  d_psi_d_SG_D_13_block : Subsystem
  d_psi_fd_SG_D_13_block : Subsystem
  d_psi_gq_SG_D_13_block : Subsystem
  d_psi_kq_SG_D_13_block : Subsystem
  d_psi_q_SG_D_13_block : Subsystem
  d_theta_SG_D_13_block : Subsystem
  d_w_SG_D_13_block : Subsystem
  i_d_SG_D_13_block : Subsystem
  i_q_SG_D_13_block : Subsystem
  psi_1d_SG_D_13 : Integrator  InitialCondition=0.9350555244258525
  psi_d_SG_D_13 : Integrator  InitialCondition=0.9226722351052147
  psi_fd_SG_D_13 : Integrator  InitialCondition=0.9974673026018663
  psi_gq_SG_D_13 : Integrator  InitialCondition=0.23792494987729754
  psi_kq_SG_D_13 : Integrator  InitialCondition=-0.3717577341832774
  psi_q_SG_D_13 : Integrator  InitialCondition=-0.38662804355060854
  theta_SG_D_13 : Integrator  InitialCondition=0.4224442384242141
  theta_SG_D_13_out_block : Subsystem
  w_SG_D_13 : Integrator  InitialCondition=376.99111843077515
  w_SG_D_13_out_block : Subsystem
  i_d_SG_D_13 : Outport
  i_q_SG_D_13 : Outport  Port=2
  T_e_SG_D_13 : Outport  Port=3
  w_SG_D_13_out : Outport  Port=4
  theta_SG_D_13_out : Outport  Port=5
  wires:
  w_SG_D_13/1 -> d_psi_q_SG_D_13_block/9(State_w_SG_D_13_af3fa), d_psi_d_SG_D_13_block/9(State_w_SG_D_13_602e4), d_w_SG_D_13_block/1(State_w_SG_D_13_19ab7), d_V_f_SG_D_13_block/8(State_w_SG_D_13_84e7f), d_V_f_SG_D_13_block/13(State_w_SG_D_13_6f79b), d_theta_SG_D_13_block/1(State_w_SG_D_13_8eb78), d_Px_1_SG_D_13_block/2(State_w_SG_D_13_74c4a), d_Px_2_SG_D_13_block/4(State_w_SG_D_13_e5bee), d_Px_3_SG_D_13_block/6(State_w_SG_D_13_2383e), w_SG_D_13_out_block/1(State_w_SG_D_13_75d42), d_T_m_SG_D_13_block/1(State_w_SG_D_13_0a956)
  d_w_SG_D_13_block/1(Blockout_d_w_SG_D_13_b8f6b) -> w_SG_D_13/1
  w_SG_D_13_out_block/1(Blockout_w_SG_D_13_out_dacbe) -> w_SG_D_13_out/1
  d_theta_SG_D_13_block/1(Blockout_d_theta_SG_D_13_8df5a) -> theta_SG_D_13/1
  d_E_fd_SG_D_13_block/1(Blockout_d_E_fd_SG_D_13_44364) -> E_fd_SG_D_13/1
  psi_gq_SG_D_13/1 -> d_psi_q_SG_D_13_block/1(State_psi_gq_SG_D_13_b9e70), d_psi_gq_SG_D_13_block/2(State_psi_gq_SG_D_13_12a06), d_psi_gq_SG_D_13_block/4(State_psi_gq_SG_D_13_9dfd7), d_psi_kq_SG_D_13_block/1(State_psi_gq_SG_D_13_cdb7e), d_psi_gq_SG_D_13_block/7(State_psi_gq_SG_D_13_f8d15), d_w_SG_D_13_block/4(State_psi_gq_SG_D_13_70bd9), d_V_f_SG_D_13_block/9(State_psi_gq_SG_D_13_2ec25), i_d_SG_D_13_block/1(State_psi_gq_SG_D_13_121f4), d_psi_kq_SG_D_13_block/3(State_psi_gq_SG_D_13_0b0ed), i_q_SG_D_13_block/1(State_psi_gq_SG_D_13_381c7), T_e_SG_D_13_block/2(State_psi_gq_SG_D_13_e02fa), d_psi_gq_SG_D_13_block/1(State_psi_gq_SG_D_13_d26d2)
  d_Px_1_SG_D_13_block/1(Blockout_d_Px_1_SG_D_13_d2c91) -> Px_1_SG_D_13/1
  d_Px_3_SG_D_13_block/1(Blockout_d_Px_3_SG_D_13_010ed) -> Px_3_SG_D_13/1
  d_T_m_SG_D_13_block/1(Blockout_d_T_m_SG_D_13_01371) -> T_m_SG_D_13/1
  d_Px_2_SG_D_13_block/1(Blockout_d_Px_2_SG_D_13_f64fc) -> Px_2_SG_D_13/1
  psi_kq_SG_D_13/1 -> d_psi_q_SG_D_13_block/2(State_psi_kq_SG_D_13_777e8), d_psi_gq_SG_D_13_block/3(State_psi_kq_SG_D_13_0827f), d_psi_gq_SG_D_13_block/5(State_psi_kq_SG_D_13_78acb), d_psi_kq_SG_D_13_block/4(State_psi_kq_SG_D_13_80acc), d_psi_kq_SG_D_13_block/2(State_psi_kq_SG_D_13_cfe97), d_w_SG_D_13_block/5(State_psi_kq_SG_D_13_63ece), d_V_f_SG_D_13_block/10(State_psi_kq_SG_D_13_bc5c2), i_q_SG_D_13_block/2(State_psi_kq_SG_D_13_c3f80), i_d_SG_D_13_block/2(State_psi_kq_SG_D_13_7664a), d_psi_gq_SG_D_13_block/8(State_psi_kq_SG_D_13_7423f), T_e_SG_D_13_block/3(State_psi_kq_SG_D_13_3f4a0)
  psi_d_SG_D_13/1 -> d_psi_fd_SG_D_13_block/6(State_psi_d_SG_D_13_f5341), d_psi_d_SG_D_13_block/2(State_psi_d_SG_D_13_8aacd), d_psi_q_SG_D_13_block/8(State_psi_d_SG_D_13_acca0), d_psi_1d_SG_D_13_block/4(State_psi_d_SG_D_13_069ec), d_w_SG_D_13_block/3(State_psi_d_SG_D_13_11de5), d_V_f_SG_D_13_block/5(State_psi_d_SG_D_13_820bf), d_psi_fd_SG_D_13_block/9(State_psi_d_SG_D_13_8fa6c), d_V_f_SG_D_13_block/12(State_psi_d_SG_D_13_11e39), i_d_SG_D_13_block/6(State_psi_d_SG_D_13_e9088), i_q_SG_D_13_block/6(State_psi_d_SG_D_13_cb45e), T_e_SG_D_13_block/1(State_psi_d_SG_D_13_06e9a), d_w_SG_D_13_block/9(State_psi_d_SG_D_13_5219f), T_e_SG_D_13_block/7(State_psi_d_SG_D_13_1b221)
  v_q_SG_D_13/1 -> d_psi_d_SG_D_13_block/6(Input_v_q_SG_D_13_58b42), d_psi_q_SG_D_13_block/6(Input_v_q_SG_D_13_89396)
  v_d_SG_D_13/1 -> d_psi_q_SG_D_13_block/4(Input_v_d_SG_D_13_60103), d_psi_d_SG_D_13_block/4(Input_v_d_SG_D_13_b2974)
  theta_SG_D_13/1 -> d_psi_d_SG_D_13_block/5(State_theta_SG_D_13_2e399), d_psi_d_SG_D_13_block/7(State_theta_SG_D_13_2b5b0), i_d_SG_D_13_block/4(State_theta_SG_D_13_1a75b), i_q_SG_D_13_block/4(State_theta_SG_D_13_aa038), d_psi_q_SG_D_13_block/5(State_theta_SG_D_13_d73b7), i_q_SG_D_13_block/8(State_theta_SG_D_13_016c8), i_d_SG_D_13_block/8(State_theta_SG_D_13_6f0a0), d_psi_q_SG_D_13_block/7(State_theta_SG_D_13_d24c4), theta_SG_D_13_out_block/1(State_theta_SG_D_13_4a098)
  T_m_SG_D_13/1 -> d_w_SG_D_13_block/2(State_T_m_SG_D_13_4085f), d_T_m_SG_D_13_block/2(State_T_m_SG_D_13_e67bf)
  Px_1_SG_D_13/1 -> d_Px_2_SG_D_13_block/2(State_Px_1_SG_D_13_fc4bf), d_Px_2_SG_D_13_block/3(State_Px_1_SG_D_13_6d859), d_Px_3_SG_D_13_block/4(State_Px_1_SG_D_13_828dc), d_Px_1_SG_D_13_block/1(State_Px_1_SG_D_13_cb051), d_Px_3_SG_D_13_block/5(State_Px_1_SG_D_13_42a56)
  Px_2_SG_D_13/1 -> d_Px_2_SG_D_13_block/1(State_Px_2_SG_D_13_19d18), d_Px_3_SG_D_13_block/3(State_Px_2_SG_D_13_0dea7), d_Px_3_SG_D_13_block/2(State_Px_2_SG_D_13_30d9f)
  Px_3_SG_D_13/1 -> d_V_f_SG_D_13_block/3(State_Px_3_SG_D_13_a1130), d_Px_3_SG_D_13_block/1(State_Px_3_SG_D_13_880e6)
  psi_q_SG_D_13/1 -> d_psi_d_SG_D_13_block/8(State_psi_q_SG_D_13_c4468), d_psi_gq_SG_D_13_block/6(State_psi_q_SG_D_13_40583), d_psi_gq_SG_D_13_block/9(State_psi_q_SG_D_13_9a89d), d_psi_q_SG_D_13_block/3(State_psi_q_SG_D_13_352e5), d_psi_kq_SG_D_13_block/5(State_psi_q_SG_D_13_4239b), d_V_f_SG_D_13_block/7(State_psi_q_SG_D_13_72752), d_V_f_SG_D_13_block/11(State_psi_q_SG_D_13_3ca0e), d_w_SG_D_13_block/7(State_psi_q_SG_D_13_4a816), i_q_SG_D_13_block/3(State_psi_q_SG_D_13_b9242), T_e_SG_D_13_block/4(State_psi_q_SG_D_13_bdd94), i_d_SG_D_13_block/3(State_psi_q_SG_D_13_649a2), d_w_SG_D_13_block/6(State_psi_q_SG_D_13_5c293), T_e_SG_D_13_block/5(State_psi_q_SG_D_13_99ec5)
  psi_1d_SG_D_13/1 -> d_psi_d_SG_D_13_block/1(State_psi_1d_SG_D_13_9b112), d_psi_1d_SG_D_13_block/3(State_psi_1d_SG_D_13_b86a3), d_V_f_SG_D_13_block/4(State_psi_1d_SG_D_13_50567), d_psi_1d_SG_D_13_block/1(State_psi_1d_SG_D_13_5ea9c), d_w_SG_D_13_block/8(State_psi_1d_SG_D_13_7983e), i_d_SG_D_13_block/5(State_psi_1d_SG_D_13_cb17c), d_psi_fd_SG_D_13_block/3(State_psi_1d_SG_D_13_e35eb), d_psi_fd_SG_D_13_block/8(State_psi_1d_SG_D_13_4aa56), i_q_SG_D_13_block/5(State_psi_1d_SG_D_13_71e2a), d_psi_fd_SG_D_13_block/5(State_psi_1d_SG_D_13_2bb65), T_e_SG_D_13_block/6(State_psi_1d_SG_D_13_43b2f)
  psi_fd_SG_D_13/1 -> d_psi_fd_SG_D_13_block/2(State_psi_fd_SG_D_13_37be0), d_psi_fd_SG_D_13_block/4(State_psi_fd_SG_D_13_e705d), d_psi_fd_SG_D_13_block/7(State_psi_fd_SG_D_13_f9d12), d_psi_fd_SG_D_13_block/10(State_psi_fd_SG_D_13_a6df8), d_psi_d_SG_D_13_block/3(State_psi_fd_SG_D_13_f7d01), d_psi_1d_SG_D_13_block/2(State_psi_fd_SG_D_13_02d25), d_w_SG_D_13_block/10(State_psi_fd_SG_D_13_7ff7c), d_V_f_SG_D_13_block/6(State_psi_fd_SG_D_13_f6a9e), i_q_SG_D_13_block/7(State_psi_fd_SG_D_13_eeae7), T_e_SG_D_13_block/8(State_psi_fd_SG_D_13_b4f3b), i_d_SG_D_13_block/7(State_psi_fd_SG_D_13_9dba0), d_psi_1d_SG_D_13_block/5(State_psi_fd_SG_D_13_cf913)
  d_R_f_SG_D_13_block/1(Blockout_d_R_f_SG_D_13_a8827) -> R_f_SG_D_13/1
  d_psi_d_SG_D_13_block/1(Blockout_d_psi_d_SG_D_13_069d2) -> psi_d_SG_D_13/1
  theta_SG_D_13_out_block/1(Blockout_theta_SG_D_13_out_b8705) -> theta_SG_D_13_out/1
  d_V_f_SG_D_13_block/1(Blockout_d_V_f_SG_D_13_c6c4a) -> V_f_SG_D_13/1
  i_d_SG_D_13_block/1(Blockout_i_d_SG_D_13_47119) -> i_d_SG_D_13/1
  T_e_SG_D_13_block/1(Blockout_T_e_SG_D_13_a0e2b) -> T_e_SG_D_13/1
  i_q_SG_D_13_block/1(Blockout_i_q_SG_D_13_d5b5c) -> i_q_SG_D_13/1
  d_psi_kq_SG_D_13_block/1(Blockout_d_psi_kq_SG_D_13_a0846) -> psi_kq_SG_D_13/1
  d_psi_gq_SG_D_13_block/1(Blockout_d_psi_gq_SG_D_13_d3799) -> psi_gq_SG_D_13/1
  d_psi_q_SG_D_13_block/1(Blockout_d_psi_q_SG_D_13_271e8) -> psi_q_SG_D_13/1
  d_psi_1d_SG_D_13_block/1(Blockout_d_psi_1d_SG_D_13_abf30) -> psi_1d_SG_D_13/1
  E_fd_SG_D_13/1 -> d_V_f_SG_D_13_block/1(State_E_fd_SG_D_13_836d5), d_R_f_SG_D_13_block/1(State_E_fd_SG_D_13_3beb5), d_psi_fd_SG_D_13_block/1(State_E_fd_SG_D_13_51a5d), d_E_fd_SG_D_13_block/1(State_E_fd_SG_D_13_5a679)
  R_f_SG_D_13/1 -> d_V_f_SG_D_13_block/2(State_R_f_SG_D_13_41787), d_R_f_SG_D_13_block/2(State_R_f_SG_D_13_66dca)
  V_f_SG_D_13/1 -> d_V_f_SG_D_13_block/14(State_V_f_SG_D_13_e839d), d_E_fd_SG_D_13_block/2(State_V_f_SG_D_13_6d482)
  d_psi_fd_SG_D_13_block/1(Blockout_d_psi_fd_SG_D_13_87f69) -> psi_fd_SG_D_13/1

== system IEEE30_case/SG_D_2 ==
  v_d_SG_D_2 : Inport
  v_q_SG_D_2 : Inport  Port=2
  E_fd_SG_D_2 : Integrator  InitialCondition=1.96926579734704
  Px_1_SG_D_2 : Integrator  InitialCondition=0.0
  Px_2_SG_D_2 : Integrator  InitialCondition=0.0
  Px_3_SG_D_2 : Integrator  InitialCondition=-5.355019995916394e-29
  R_f_SG_D_2 : Integrator  InitialCondition=13.295357368945874
  T_e_SG_D_2_block : Subsystem
  T_m_SG_D_2 : Integrator  InitialCondition=0.6102158508039623
  V_f_SG_D_2 : Integrator  InitialCondition=19.6926579734704
  d_E_fd_SG_D_2_block : Subsystem
  d_Px_1_SG_D_2_block : Subsystem
  d_Px_2_SG_D_2_block : Subsystem
  d_Px_3_SG_D_2_block : Subsystem
  d_R_f_SG_D_2_block : Subsystem
  d_T_m_SG_D_2_block : Subsystem
  d_V_f_SG_D_2_block : Subsystem
  d_psi_1d_SG_D_2_block : Subsystem
  d_psi_d_SG_D_2_block : Subsystem
  d_psi_fd_SG_D_2_block : Subsystem
  d_psi_gq_SG_D_2_block : Subsystem
  d_psi_kq_SG_D_2_block : Subsystem
  d_psi_q_SG_D_2_block : Subsystem
  d_theta_SG_D_2_block : Subsystem
  d_w_SG_D_2_block : Subsystem
  i_d_SG_D_2_block : Subsystem
  i_q_SG_D_2_block : Subsystem
  psi_1d_SG_D_2 : Integrator  InitialCondition=0.9020378890619168
  psi_d_SG_D_2 : Integrator  InitialCondition=0.8731938915406972
  psi_fd_SG_D_2 : Integrator  InitialCondition=1.0474116365688635
  psi_gq_SG_D_2 : Integrator  InitialCondition=0.30075861241991825
  psi_kq_SG_D_2 : Integrator  InitialCondition=-0.4699353319061223
  psi_q_SG_D_2 : Integrator  InitialCondition=-0.48873274518236715
  theta_SG_D_2 : Integrator  InitialCondition=0.5026656539335864
  theta_SG_D_2_out_block : Subsystem
  w_SG_D_2 : Integrator  InitialCondition=376.99111843077515
  w_SG_D_2_out_block : Subsystem
  i_d_SG_D_2 : Outport
  i_q_SG_D_2 : Outport  Port=2
  T_e_SG_D_2 : Outport  Port=3
  w_SG_D_2_out : Outport  Port=4
  theta_SG_D_2_out : Outport  Port=5
  wires:
  d_T_m_SG_D_2_block/1(Blockout_d_T_m_SG_D_2_a9295) -> T_m_SG_D_2/1
  T_e_SG_D_2_block/1(Blockout_T_e_SG_D_2_01d05) -> T_e_SG_D_2/1
  d_Px_2_SG_D_2_block/1(Blockout_d_Px_2_SG_D_2_fe4d9) -> Px_2_SG_D_2/1
  w_SG_D_2/1 -> d_psi_d_SG_D_2_block/9(State_w_SG_D_2_cc748), d_w_SG_D_2_block/1(State_w_SG_D_2_071c4), d_V_f_SG_D_2_block/13(State_w_SG_D_2_49a6f), d_T_m_SG_D_2_block/1(State_w_SG_D_2_b536b), d_psi_q_SG_D_2_block/9(State_w_SG_D_2_5f632), d_Px_1_SG_D_2_block/2(State_w_SG_D_2_0d596), d_V_f_SG_D_2_block/8(State_w_SG_D_2_28647), d_Px_2_SG_D_2_block/4(State_w_SG_D_2_2a02e), d_theta_SG_D_2_block/1(State_w_SG_D_2_d4d26), d_Px_3_SG_D_2_block/6(State_w_SG_D_2_59107), w_SG_D_2_out_block/1(State_w_SG_D_2_6b0c6)
  psi_q_SG_D_2/1 -> d_psi_d_SG_D_2_block/8(State_psi_q_SG_D_2_54436), d_psi_q_SG_D_2_block/3(State_psi_q_SG_D_2_22b60), d_psi_gq_SG_D_2_block/6(State_psi_q_SG_D_2_83abf), d_psi_kq_SG_D_2_block/5(State_psi_q_SG_D_2_69b92), d_w_SG_D_2_block/6(State_psi_q_SG_D_2_76d6b), d_V_f_SG_D_2_block/7(State_psi_q_SG_D_2_9610e), i_d_SG_D_2_block/3(State_psi_q_SG_D_2_14a65), d_V_f_SG_D_2_block/11(State_psi_q_SG_D_2_6a31d), d_w_SG_D_2_block/7(State_psi_q_SG_D_2_b0e4a), d_psi_gq_SG_D_2_block/9(State_psi_q_SG_D_2_6cd36), T_e_SG_D_2_block/4(State_psi_q_SG_D_2_2791a), T_e_SG_D_2_block/5(State_psi_q_SG_D_2_b8bd3), i_q_SG_D_2_block/3(State_psi_q_SG_D_2_c9d02)
  w_SG_D_2_out_block/1(Blockout_w_SG_D_2_out_ca3f3) -> w_SG_D_2_out/1
  d_Px_1_SG_D_2_block/1(Blockout_d_Px_1_SG_D_2_215fb) -> Px_1_SG_D_2/1
  d_theta_SG_D_2_block/1(Blockout_d_theta_SG_D_2_cbd9d) -> theta_SG_D_2/1
  d_Px_3_SG_D_2_block/1(Blockout_d_Px_3_SG_D_2_f118f) -> Px_3_SG_D_2/1
  psi_gq_SG_D_2/1 -> d_psi_q_SG_D_2_block/1(State_psi_gq_SG_D_2_77760), d_psi_gq_SG_D_2_block/1(State_psi_gq_SG_D_2_104a2), d_psi_gq_SG_D_2_block/7(State_psi_gq_SG_D_2_e51c7), d_w_SG_D_2_block/4(State_psi_gq_SG_D_2_9f73e), d_V_f_SG_D_2_block/9(State_psi_gq_SG_D_2_6dc45), d_psi_kq_SG_D_2_block/3(State_psi_gq_SG_D_2_5ea4a), d_psi_gq_SG_D_2_block/2(State_psi_gq_SG_D_2_afe73), i_d_SG_D_2_block/1(State_psi_gq_SG_D_2_ef87c), T_e_SG_D_2_block/2(State_psi_gq_SG_D_2_e2d2d), i_q_SG_D_2_block/1(State_psi_gq_SG_D_2_0f140), d_psi_gq_SG_D_2_block/4(State_psi_gq_SG_D_2_1bb75), d_psi_kq_SG_D_2_block/1(State_psi_gq_SG_D_2_68a38)
  psi_kq_SG_D_2/1 -> d_psi_q_SG_D_2_block/2(State_psi_kq_SG_D_2_d2951), d_psi_gq_SG_D_2_block/3(State_psi_kq_SG_D_2_5e865), d_psi_gq_SG_D_2_block/8(State_psi_kq_SG_D_2_7a2a4), d_psi_kq_SG_D_2_block/4(State_psi_kq_SG_D_2_73d66), d_psi_kq_SG_D_2_block/2(State_psi_kq_SG_D_2_4ef7d), d_psi_gq_SG_D_2_block/5(State_psi_kq_SG_D_2_721d7), d_V_f_SG_D_2_block/10(State_psi_kq_SG_D_2_f6f79), i_q_SG_D_2_block/2(State_psi_kq_SG_D_2_8caff), i_d_SG_D_2_block/2(State_psi_kq_SG_D_2_da414), T_e_SG_D_2_block/3(State_psi_kq_SG_D_2_b5b81), d_w_SG_D_2_block/5(State_psi_kq_SG_D_2_c590e)
  theta_SG_D_2/1 -> d_psi_d_SG_D_2_block/5(State_theta_SG_D_2_7fad9), d_psi_d_SG_D_2_block/7(State_theta_SG_D_2_809cf), i_d_SG_D_2_block/4(State_theta_SG_D_2_b0b05), i_d_SG_D_2_block/8(State_theta_SG_D_2_57fa8), d_psi_q_SG_D_2_block/7(State_theta_SG_D_2_018ce), d_psi_q_SG_D_2_block/5(State_theta_SG_D_2_05bbc), i_q_SG_D_2_block/8(State_theta_SG_D_2_e3ac6), theta_SG_D_2_out_block/1(State_theta_SG_D_2_1ecf4), i_q_SG_D_2_block/4(State_theta_SG_D_2_99776)
  v_d_SG_D_2/1 -> d_psi_d_SG_D_2_block/4(Input_v_d_SG_D_2_98b6e), d_psi_q_SG_D_2_block/4(Input_v_d_SG_D_2_67bf0)
  d_V_f_SG_D_2_block/1(Blockout_d_V_f_SG_D_2_9f874) -> V_f_SG_D_2/1
  v_q_SG_D_2/1 -> d_psi_d_SG_D_2_block/6(Input_v_q_SG_D_2_5c158), d_psi_q_SG_D_2_block/6(Input_v_q_SG_D_2_2e6d8)
  Px_1_SG_D_2/1 -> d_Px_1_SG_D_2_block/1(State_Px_1_SG_D_2_b4144), d_Px_2_SG_D_2_block/2(State_Px_1_SG_D_2_4e32d), d_Px_2_SG_D_2_block/3(State_Px_1_SG_D_2_8c524), d_Px_3_SG_D_2_block/4(State_Px_1_SG_D_2_7331f), d_Px_3_SG_D_2_block/5(State_Px_1_SG_D_2_9d5b2)
  T_m_SG_D_2/1 -> d_T_m_SG_D_2_block/2(State_T_m_SG_D_2_c8c02), d_w_SG_D_2_block/2(State_T_m_SG_D_2_860e5)
  i_d_SG_D_2_block/1(Blockout_i_d_SG_D_2_ae2df) -> i_d_SG_D_2/1
  psi_d_SG_D_2/1 -> d_psi_fd_SG_D_2_block/6(State_psi_d_SG_D_2_4b3f7), d_psi_fd_SG_D_2_block/9(State_psi_d_SG_D_2_ea571), d_psi_d_SG_D_2_block/2(State_psi_d_SG_D_2_ba6c1), d_psi_q_SG_D_2_block/8(State_psi_d_SG_D_2_4e236), d_psi_1d_SG_D_2_block/4(State_psi_d_SG_D_2_140c5), d_w_SG_D_2_block/9(State_psi_d_SG_D_2_9b8cf), d_V_f_SG_D_2_block/12(State_psi_d_SG_D_2_a1417), d_w_SG_D_2_block/3(State_psi_d_SG_D_2_34ede), i_d_SG_D_2_block/6(State_psi_d_SG_D_2_956af), i_q_SG_D_2_block/6(State_psi_d_SG_D_2_82684), T_e_SG_D_2_block/1(State_psi_d_SG_D_2_5c155), d_V_f_SG_D_2_block/5(State_psi_d_SG_D_2_13dc4), T_e_SG_D_2_block/7(State_psi_d_SG_D_2_c3c7e)
  psi_1d_SG_D_2/1 -> d_psi_fd_SG_D_2_block/3(State_psi_1d_SG_D_2_36843), d_psi_fd_SG_D_2_block/5(State_psi_1d_SG_D_2_42d8b), d_psi_fd_SG_D_2_block/8(State_psi_1d_SG_D_2_a65ff), d_psi_d_SG_D_2_block/1(State_psi_1d_SG_D_2_df2dd), d_psi_1d_SG_D_2_block/3(State_psi_1d_SG_D_2_ea3e5), d_psi_1d_SG_D_2_block/1(State_psi_1d_SG_D_2_46e59), d_w_SG_D_2_block/8(State_psi_1d_SG_D_2_97ed5), d_V_f_SG_D_2_block/4(State_psi_1d_SG_D_2_a974f), i_d_SG_D_2_block/5(State_psi_1d_SG_D_2_baa39), i_q_SG_D_2_block/5(State_psi_1d_SG_D_2_3670e), T_e_SG_D_2_block/6(State_psi_1d_SG_D_2_ae46f)
  Px_2_SG_D_2/1 -> d_Px_2_SG_D_2_block/1(State_Px_2_SG_D_2_06380), d_Px_3_SG_D_2_block/2(State_Px_2_SG_D_2_f8442), d_Px_3_SG_D_2_block/3(State_Px_2_SG_D_2_0d955)
  psi_fd_SG_D_2/1 -> d_psi_fd_SG_D_2_block/2(State_psi_fd_SG_D_2_a9693), d_psi_fd_SG_D_2_block/4(State_psi_fd_SG_D_2_74282), d_psi_fd_SG_D_2_block/7(State_psi_fd_SG_D_2_d0da0), d_psi_fd_SG_D_2_block/10(State_psi_fd_SG_D_2_33a5d), d_psi_d_SG_D_2_block/3(State_psi_fd_SG_D_2_fffbd), d_psi_1d_SG_D_2_block/5(State_psi_fd_SG_D_2_f6724), d_w_SG_D_2_block/10(State_psi_fd_SG_D_2_66d61), d_V_f_SG_D_2_block/6(State_psi_fd_SG_D_2_f4996), i_d_SG_D_2_block/7(State_psi_fd_SG_D_2_52aed), d_psi_1d_SG_D_2_block/2(State_psi_fd_SG_D_2_4eec5), i_q_SG_D_2_block/7(State_psi_fd_SG_D_2_4cfda), T_e_SG_D_2_block/8(State_psi_fd_SG_D_2_fdba3)
  R_f_SG_D_2/1 -> d_V_f_SG_D_2_block/2(State_R_f_SG_D_2_2963a), d_R_f_SG_D_2_block/2(State_R_f_SG_D_2_6571e)
  theta_SG_D_2_out_block/1(Blockout_theta_SG_D_2_out_e958d) -> theta_SG_D_2_out/1
  d_psi_gq_SG_D_2_block/1(Blockout_d_psi_gq_SG_D_2_e9d2a) -> psi_gq_SG_D_2/1
  d_psi_kq_SG_D_2_block/1(Blockout_d_psi_kq_SG_D_2_68567) -> psi_kq_SG_D_2/1
  d_psi_q_SG_D_2_block/1(Blockout_d_psi_q_SG_D_2_4be96) -> psi_q_SG_D_2/1
  d_R_f_SG_D_2_block/1(Blockout_d_R_f_SG_D_2_b95c5) -> R_f_SG_D_2/1
  i_q_SG_D_2_block/1(Blockout_i_q_SG_D_2_865bf) -> i_q_SG_D_2/1
  d_w_SG_D_2_block/1(Blockout_d_w_SG_D_2_6b1c2) -> w_SG_D_2/1
  d_psi_d_SG_D_2_block/1(Blockout_d_psi_d_SG_D_2_e4800) -> psi_d_SG_D_2/1
  d_psi_1d_SG_D_2_block/1(Blockout_d_psi_1d_SG_D_2_b4ac5) -> psi_1d_SG_D_2/1
  Px_3_SG_D_2/1 -> d_Px_3_SG_D_2_block/1(State_Px_3_SG_D_2_dac62), d_V_f_SG_D_2_block/3(State_Px_3_SG_D_2_48694)
  V_f_SG_D_2/1 -> d_E_fd_SG_D_2_block/2(State_V_f_SG_D_2_b9fa9), d_V_f_SG_D_2_block/14(State_V_f_SG_D_2_edaff)
  d_E_fd_SG_D_2_block/1(Blockout_d_E_fd_SG_D_2_39068) -> E_fd_SG_D_2/1
  E_fd_SG_D_2/1 -> d_V_f_SG_D_2_block/1(State_E_fd_SG_D_2_07148), d_E_fd_SG_D_2_block/1(State_E_fd_SG_D_2_d1f2e), d_R_f_SG_D_2_block/1(State_E_fd_SG_D_2_d5c8d), d_psi_fd_SG_D_2_block/1(State_E_fd_SG_D_2_9e073)
  d_psi_fd_SG_D_2_block/1(Blockout_d_psi_fd_SG_D_2_9f80c) -> psi_fd_SG_D_2/1
